simulink model "guide01"  (Simulink 7.2)
settings: Solver=FixedStepDiscrete  StartTime=0.0  StopTime=inf  RelTol=1e-3
InitFcn:
  | godiva_initfcn('tal')
libraries: simulink x3
settings Model: Creator=alfnie  LastModifiedBy=alfnie
settings OptimizationCC: BlockReduction=off
settings DebuggingCC: UnconnectedInputMsg=none  UnconnectedOutputMsg=none  UnconnectedLineMsg=none

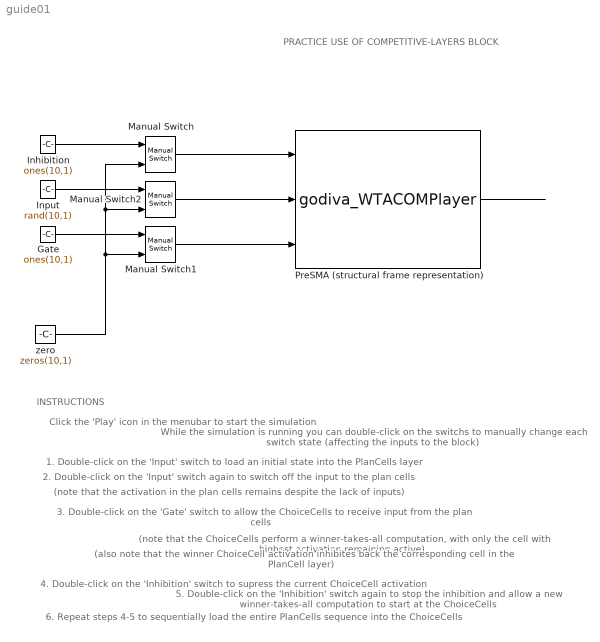
== system guide01 ==
  note: INSTRUCTIONS
  note: Click the 'Play' icon in the menubar to start the simulation
  note: PRACTICE USE OF COMPETITIVE-LAYERS BLOCK
  note: While the simulation is running you can double-click on the switchs to manually change each switch state (affecting the inputs to the block)
  note: 1. Double-click on the 'Input' switch to load an initial state into the PlanCells layer
  note: 2. Double-click on the 'Input' switch again to switch off the input to the plan cells
  note: 3. Double-click on the 'Gate' switch to allow the ChoiceCells to receive input from the plan cells
  note: (note that the ChoiceCells perform a winner-takes-all computation, with only the cell with highest activation remaining active)
  note: (also note that the winner ChoiceCell activation inhibites back the corresponding cell in the PlanCell layer)
  note: (note that the activation in the plan cells remains despite the lack of inputs)
  note: 4. Double-click on the 'Inhibition' switch to supress the current ChoiceCell activation
  note: 5. Double-click on the 'Inhibition' switch again to stop the inhibition and allow a new winner-takes-all computation to start at the ChoiceCells
  note: 6. Repeat steps 4-5 to sequentially load the entire PlanCells sequence into the ChoiceCells
  Gate : Constant  Value=ones(10,1)  OutDataType=sfix(16)  OutScaling=2^0  SampleTime=.001
  Inhibition : Constant  Value=ones(10,1)  OutDataType=sfix(16)  OutScaling=2^0  SampleTime=.001
  Input : Constant  Value=rand(10,1)  OutDataType=sfix(16)  OutScaling=2^0  SampleTime=.001
  Manual Switch : simulink/Signal Routing/Manual Switch  SystemSampleTime=-1  sw=0  action=0  varsize=off
  Manual Switch1 : simulink/Signal Routing/Manual Switch  SystemSampleTime=-1  sw=0  action=0  varsize=off
  Manual Switch2 : simulink/Signal Routing/Manual Switch  SystemSampleTime=-1  sw=0  action=0  varsize=off
  PreSMA (structural frame representation) : M-S-Function  FunctionName=godiva_WTACOMPlayer  Parameters='PreSMA', 1 , 0, 1
      mask Description: Plan / Choice competitive layer
      mask Display: image(imread('godiva_WTAlayer01.jpg'))
  zero : Constant  Value=zeros(10,1)  OutDataType=sfix(16)  OutScaling=2^0
  wires:
  Manual Switch/1 -> PreSMA (structural frame representation)/1
  Manual Switch2/1 -> PreSMA (structural frame representation)/2
  Manual Switch1/1 -> PreSMA (structural frame representation)/3
  PreSMA (structural frame representation)/1 -> ?
  Inhibition/1 -> Manual Switch/1
  zero/1 -> Manual Switch1/2, Manual Switch2/2, Manual Switch/2
  Input/1 -> Manual Switch2/1
  Gate/1 -> Manual Switch1/1
